simulink model "L1AC_test2_design_and_analysis_2008"  (R2018b)
settings: Solver=ode14x  StartTime=0.0  StopTime=100  FixedStep=0.001  RelTol=1e-3
undefined symbols (not defined in the file or in its folder): kt, thet1o, thet2o
libraries: simulink x1
settings Model: Creator=Jcong  LastModifiedBy=Jcong

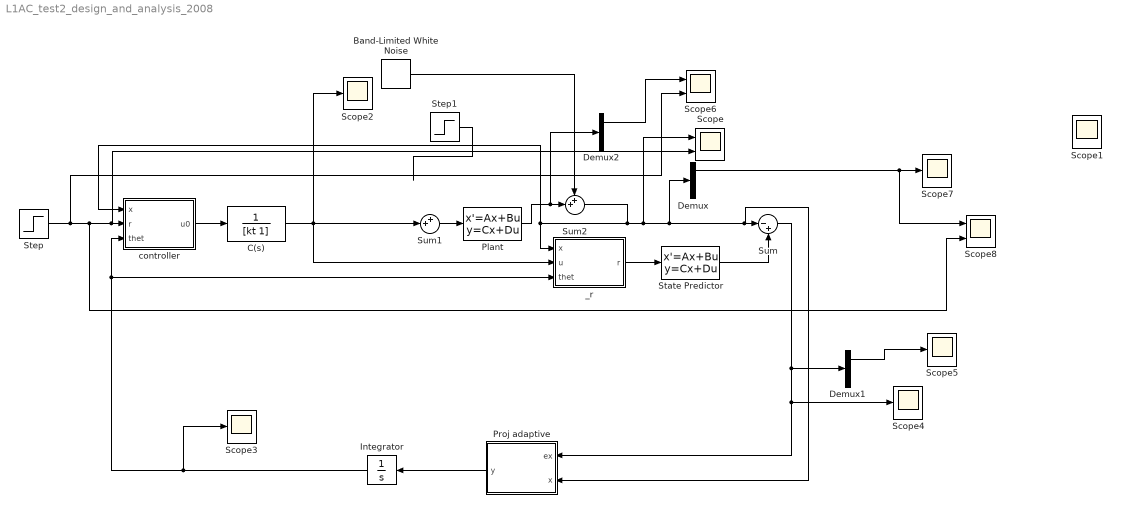
== system L1AC_test2_design_and_analysis_2008 ==
  Band-Limited White Noise : simulink/Sources/Band-Limited White Noise  Cov=[0.000001]  Ts=0.001  seed=[23341]
  C(s) : TransferFcn  Denominator=[kt 1]
  Demux : Demux  Outputs=2
  Demux1 : Demux  Outputs=2
  Demux2 : Demux  Outputs=2
  Integrator : Integrator
  Plant : StateSpace  A=[0,1;(-1-thet1o),(-1.4-thet2o)]  B=[0;1]  C=[1,0;0,1]  D=[0;0]  InitialCondition=[0;0]
  Proj adaptive : MATLAB Function  TreatAsAtomicUnit=on
  Scope : Scope  NumInputPorts=2
  Scope{1..5,7} (6 alike) : Scope
  Scope6 : Scope  NumInputPorts=2
  Scope8 : Scope  NumInputPorts=2
  State Predictor : StateSpace  A=[0,1;-1,-1.4]  B=[0;1]  C=[1,0;0,1]  D=[0;0]  InitialCondition=[0;0]
  Step : Step  Time=0  SampleTime=0
  Step1 : Step  Time=10  After=100  SampleTime=0
  Sum : Sum  Inputs=|-+
  Sum1 : Sum  Inputs=++|
  Sum2 : Sum  Inputs=++|
  _r : MATLAB Function  TreatAsAtomicUnit=on
  controller : MATLAB Function  TreatAsAtomicUnit=on
  wires:
  _r/1(r) -> State Predictor/1
  Sum2/1 -> controller/1(x), _r/1(x), Scope/1, Demux/1, Proj adaptive/2(x), Sum/1
  Step/1 -> Scope6/2, Scope8/2, Scope/2, controller/2(r)
  controller/1(u0) -> C(s)/1
  C(s)/1 -> Sum1/2, Scope2/1, _r/2(u)
  State Predictor/1 -> Sum/2
  Sum/1 -> Demux1/1, Scope4/1, Proj adaptive/1(ex)
  Proj adaptive/1(y) -> Integrator/1
  Integrator/1 -> Scope3/1, _r/3(thet), controller/3(thet)
  Demux/1 -> Scope8/1, Scope7/1
  Demux1/1 -> Scope5/1
  Sum1/1 -> Plant/1
  Band-Limited White Noise/1 -> Sum2/1
  Plant/1 -> Demux2/1, Sum2/2
  Step1/1 -> ?
  Demux2/1 -> Scope6/1

== matlab function L1AC_test2_design_and_analysis_2008/controller ==
  data: x input; r input; u0 output; thet input
function u0 = fcn(x,r,thet)
k=1;
u0 = thet'*x+r*k;

== matlab function L1AC_test2_design_and_analysis_2008/_r ==
  data: x input; u input; r output; thet input
function r = fcn(x,u,thet)

r = -thet'*x+u;

== matlab function L1AC_test2_design_and_analysis_2008/Proj adaptive ==
  data: ex input; y output; x input
function y = fcn(ex,x)
b=[0;1];
T=10000;
P=100;
%y =T*ex'*P*b*x;
y = T*x*ex'*P*b;
